simulink model "ProposedMIMOmodeling"  (R2020a)
settings: Solver=VariableStepAuto  StartTime=0.0  StopTime=250000  RelTol=1e-3
undefined symbols (not defined in the file): R1Kd, R1Ku, R2Kd, R2Ku, R3Kd, R3Ku
libraries: cstblocks x12
settings Model: Creator=User  LastModifiedBy=User
settings SolverCC: AlgebraicLoopSolver=LineSearch

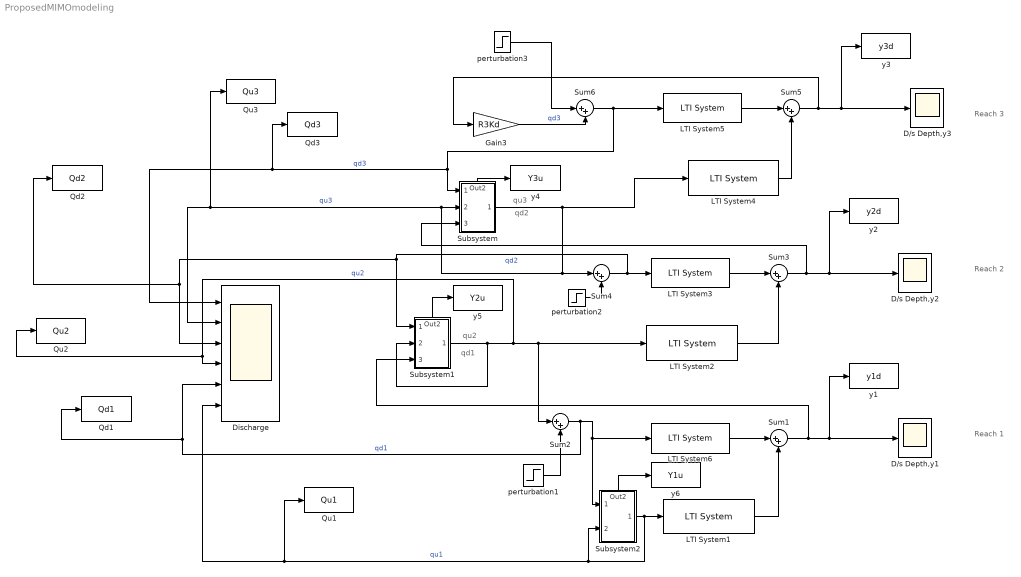
== system ProposedMIMOmodeling ==
  note: Reach 1
  note: Reach 2
  note: Reach 3
  note: qu3
  note: qu2
  note: qd2
  note: qd1
  D/s Depth,y1 : Scope
  D/s Depth,y2 : Scope
  D/s Depth,y3 : Scope
  Discharge : Scope  NumInputPorts=6
  Gain3 : Gain  Gain=R3Kd
  LTI System1 : cstblocks/LTI System  sys=R1P21  IC=[]
  LTI System2 : cstblocks/LTI System  sys=R2P21  IC=[]
  LTI System3 : cstblocks/LTI System  sys=R2P22  IC=[]
  LTI System4 : cstblocks/LTI System  sys=R3P21  IC=[]
  LTI System5 : cstblocks/LTI System  sys=R3P22  IC=[]
  LTI System6 : cstblocks/LTI System  sys=R1P22  IC=[]
  Qd1 : ToWorkspace  VariableName=Qd1  SaveFormat=Timeseries  SampleTime=-1
  Qd2 : ToWorkspace  VariableName=Qd2  SaveFormat=Timeseries  SampleTime=-1
  Qd3 : ToWorkspace  VariableName=Qd3  SaveFormat=Timeseries  SampleTime=-1
  Qu1 : ToWorkspace  VariableName=Qu1  SaveFormat=Timeseries  SampleTime=-1
  Qu2 : ToWorkspace  VariableName=Qu2  SaveFormat=Timeseries  SampleTime=-1
  Qu3 : ToWorkspace  VariableName=Qu3  SaveFormat=Timeseries  SampleTime=-1
  Subsystem : Subsystem
      settings: PortSchema="{\"entries\":[{\"content\":{\"sides\":[{\"content\":{\"connectorIds\":[\"In1\",\"In2\",\"In3\"]},\"type\":\"ConnectorPlacement.EquallySpacedRectSide\",\"uuid\":\"5966c642-27f1-4d1c-9c21-5a17e9a6fd4f\"},{\"content\":{\"connectorIds\":[\"Out1\"],\"side\":\"RIGHT\"},\"type\":\"ConnectorPlacement.EquallySpacedRectSide\",\"uuid\":\"42c3a355-b1fe-4101-8b09-079b8b81b2d6\"},{\"content\":{\"connectorIds\":[\"Out2\"],\"side\":\"TOP\"},\"type\":\"ConnectorPlacement.EquallySpacedRectSide\",\"uuid\":\"ebeefabc-9e25-4535-b836-1666cac596f0\"}]},\"type\":\"ConnectorPlacement.EquallySpacedConnector\",\"uuid\":\"256cc23c-d034-44ee-8555-a61e76b4c896\"}],\"packageUris\":[\"http://schema.mathworks.com/mf0/Connector/19700101\"],\"version\":\"1.0\"}"
  Subsystem1 : Subsystem
      settings: PortSchema="{\"entries\":[{\"content\":{\"sides\":[{\"content\":{\"connectorIds\":[\"In1\",\"In2\",\"In3\"]},\"type\":\"ConnectorPlacement.EquallySpacedRectSide\",\"uuid\":\"5966c642-27f1-4d1c-9c21-5a17e9a6fd4f\"},{\"content\":{\"connectorIds\":[\"Out1\"],\"side\":\"RIGHT\"},\"type\":\"ConnectorPlacement.EquallySpacedRectSide\",\"uuid\":\"42c3a355-b1fe-4101-8b09-079b8b81b2d6\"},{\"content\":{\"connectorIds\":[\"Out2\"],\"side\":\"TOP\"},\"type\":\"ConnectorPlacement.EquallySpacedRectSide\",\"uuid\":\"ebeefabc-9e25-4535-b836-1666cac596f0\"}]},\"type\":\"ConnectorPlacement.EquallySpacedConnector\",\"uuid\":\"256cc23c-d034-44ee-8555-a61e76b4c896\"}],\"packageUris\":[\"http://schema.mathworks.com/mf0/Connector/19700101\"],\"version\":\"1.0\"}"
  Subsystem2 : Subsystem
      settings: PortSchema="{\"entries\":[{\"content\":{\"sides\":[{\"content\":{\"connectorIds\":[\"In1\",\"In2\"]},\"type\":\"ConnectorPlacement.EquallySpacedRectSide\",\"uuid\":\"4285bcff-0b6c-4803-aa7e-52336b14ade4\"},{\"content\":{\"connectorIds\":[\"Out1\"],\"side\":\"RIGHT\"},\"type\":\"ConnectorPlacement.EquallySpacedRectSide\",\"uuid\":\"ef054825-743c-42b7-be9a-02fce2cfa877\"},{\"content\":{\"connectorIds\":[\"Out2\"],\"side\":\"TOP\"},\"type\":\"ConnectorPlacement.EquallySpacedRectSide\",\"uuid\":\"73e4ddcd-e004-417a-b0e5-3c0bfc9a3c12\"}]},\"type\":\"ConnectorPlacement.EquallySpacedConnector\",\"uuid\":\"fc460328-0800-4fc0-8c40-6130ed6b1da0\"}],\"packageUris\":[\"http://schema.mathworks.com/mf0/Connector/19700101\"],\"version\":\"1.0\"}"
  Sum{1..6} (6 alike) : Sum  Inputs=|++
  perturbation1 : Step  Time=1200  After=0  SampleTime=0
  perturbation2 : Step  Time=1200  SampleTime=0
  perturbation3 : Step  Time=1200  After=0  SampleTime=0
  y1 : ToWorkspace  VariableName=y1d  SaveFormat=Timeseries  SampleTime=-1
  y2 : ToWorkspace  VariableName=y2d  SaveFormat=Timeseries  SampleTime=-1
  y3 : ToWorkspace  VariableName=y3d  SaveFormat=Timeseries  SampleTime=-1
  y4 : ToWorkspace  VariableName=Y3u  SaveFormat=Timeseries  SampleTime=-1
  y5 : ToWorkspace  VariableName=Y2u  SaveFormat=Timeseries  SampleTime=-1
  y6 : ToWorkspace  VariableName=Y1u  SaveFormat=Timeseries  SampleTime=-1
  wires:
  LTI System3/1 -> Sum3/1
  Sum3/1 -> Subsystem/3(In3), D/s Depth,y2/1, y2/1
  LTI System2/1 -> Sum3/2
  LTI System5/1 -> Sum5/1
  perturbation3/1 -> Sum6/1
  Sum5/1 -> Gain3/1, D/s Depth,y3/1, y3/1
  Gain3/1 -> Sum6/2  "qd3"
  LTI System4/1 -> Sum5/2
  LTI System1/1 -> Sum1/2
  Subsystem2/1(Out1) -> Qu1/1, Discharge/6, Subsystem2/2(In2), LTI System1/1  "qu1"
  Sum1/1 -> Subsystem1/3(In3), D/s Depth,y1/1, y1/1
  LTI System6/1 -> Sum1/1
  Sum4/1 -> Subsystem1/1(In1), Qd2/1, Discharge/3, LTI System3/1  "qd2"
  perturbation2/1 -> Sum4/2
  Subsystem1/1(Out1) -> Qu2/1, Discharge/4, LTI System2/1, Sum2/1, Subsystem1/2(In2)  "qu2"
  perturbation1/1 -> Sum2/2
  Sum2/1 -> Qd1/1, Discharge/5, LTI System6/1, Subsystem2/1(In1)  "qd1"
  Subsystem/2(Out2) -> y4/1
  Subsystem2/2(Out2) -> y6/1
  Subsystem1/2(Out2) -> y5/1
  Subsystem/1(Out1) -> Sum4/1, Subsystem/2(In2), Qu3/1, Discharge/2, LTI System4/1  "qu3"
  Sum6/1 -> Qd3/1, Discharge/1, Subsystem/1(In1), LTI System5/1  "qd3"

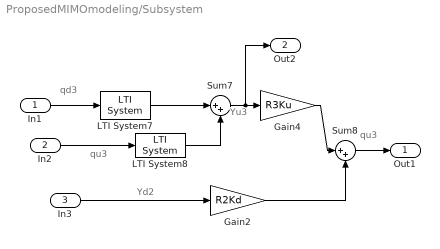
== system ProposedMIMOmodeling/Subsystem ==
  note: Yu3
  note: qd3
  note: qu3
  note: Yd2
  note: qu3
  In1 : Inport
  In2 : Inport  Port=2
  In3 : Inport  Port=3
  Gain2 : Gain  Gain=R2Kd
  Gain4 : Gain  Gain=R3Ku
  LTI System7 : cstblocks/LTI System  sys=R3P12  IC=[]
  LTI System8 : cstblocks/LTI System  sys=R3P11  IC=[]
  Sum7 : Sum  Inputs=|++
  Sum8 : Sum  Inputs=|++
  Out1 : Outport
  Out2 : Outport  Port=2
  wires:
  LTI System7/1 -> Sum7/1
  Sum7/1 -> Out2/1, Gain4/1
  Gain2/1 -> Sum8/2
  In1/1 -> LTI System7/1
  Gain4/1 -> Sum8/1
  Sum8/1 -> Out1/1
  LTI System8/1 -> Sum7/2
  In3/1 -> Gain2/1
  In2/1 -> LTI System8/1

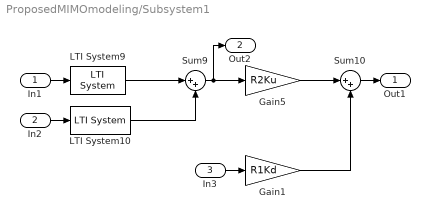
== system ProposedMIMOmodeling/Subsystem1 ==
  In1 : Inport
  In2 : Inport  Port=2
  In3 : Inport  Port=3
  Gain1 : Gain  Gain=R1Kd
  Gain5 : Gain  Gain=R2Ku
  LTI System10 : cstblocks/LTI System  sys=R2P11  IC=[]
  LTI System9 : cstblocks/LTI System  sys=R2P12  IC=[]
  Sum10 : Sum  Inputs=|++
  Sum9 : Sum  Inputs=|++
  Out1 : Outport
  Out2 : Outport  Port=2
  wires:
  LTI System9/1 -> Sum9/1
  Sum10/1 -> Out1/1
  In2/1 -> LTI System10/1
  Sum9/1 -> Out2/1, Gain5/1
  In1/1 -> LTI System9/1
  Gain5/1 -> Sum10/1
  In3/1 -> Gain1/1
  LTI System10/1 -> Sum9/2
  Gain1/1 -> Sum10/2

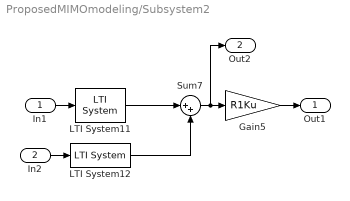
== system ProposedMIMOmodeling/Subsystem2 ==
  In1 : Inport
  In2 : Inport  Port=2
  Gain5 : Gain  Gain=R1Ku
  LTI System11 : cstblocks/LTI System  sys=R1P12  IC=[]
  LTI System12 : cstblocks/LTI System  sys=R1P11  IC=[]
  Sum7 : Sum  Inputs=|++
  Out1 : Outport
  Out2 : Outport  Port=2
  wires:
  LTI System12/1 -> Sum7/2
  Sum7/1 -> Out2/1, Gain5/1
  In1/1 -> LTI System11/1
  In2/1 -> LTI System12/1
  LTI System11/1 -> Sum7/1
  Gain5/1 -> Out1/1
